simulink model "bench"  (R2025b)
settings: Solver=ode4  StartTime=0.0  StopTime=inf  FixedStep=Ts_gcs  RelTol=1e-3
undefined symbols (not defined in the file): quadcop, Ts_gcs
libraries: instrumentseriallib x2, sldrtlib x1
settings Model: DataDictionary=project.sldd  SimulationMode=accelerator  Creator=Nick  LastModifiedBy=Rakete
settings SolverCC: AutoInsertRateTranBlk=on

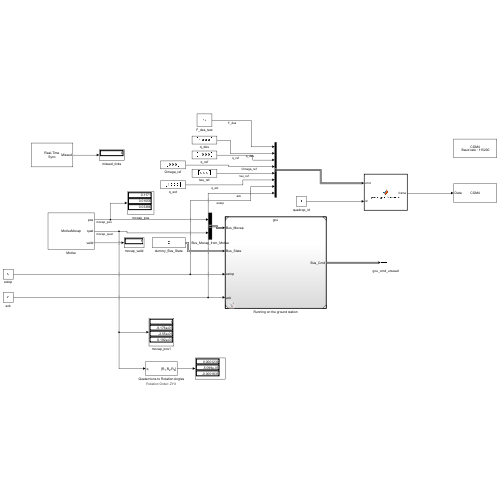
[thumbnail: Simulink's stored preview of the top-level diagram]
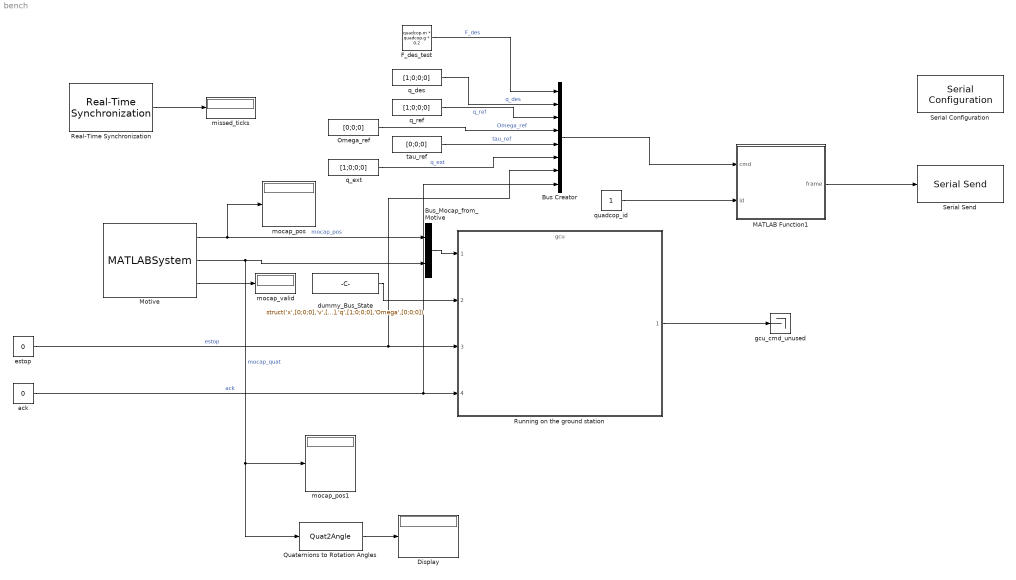
== system bench ==
  Bus Creator : BusCreator  Inputs=8  OutDataTypeStr=Bus: Bus_Cmd
  Bus_Mocap_from_Motive : BusCreator  Inputs=2  OutDataTypeStr=Bus: Bus_Mocap
  Display : Display
  F_des_test : Constant  Value=quadcop.m * quadcop.g * 0.2
  MATLAB Function1 : MATLAB Function  TreatAsAtomicUnit=on
  Motive : MATLABSystem  System=MotiveMocap  HostIP=mocap.host_ip  ClientIP=mocap.client_ip  StreamingID=mocap.streaming_id  SampleTimeSec=Ts_gcs  Verbose=on
      mask Type: MotiveMocap
  Omega_ref : Constant  Value=[0;0;0]
  Quaternions to Rotation Angles : Quat2Angle
      settings: AttributesFormatString=Rotation Order: %<rotationOrder>
  Real-Time Synchronization : sldrtlib/Real-Time Synchronization  SampleTime=Ts_gcs  MaxMissedTicks=inf  ShowMissedTicks=on  YieldWhenWaiting=off
  Running on the ground station : ModelReference  ModelNameDialog=gcu.slx  SimulationMode=Normal  ModelReferenceVersion=1.299
  Serial Configuration : instrumentseriallib/Serial Configuration  Priority=-200000  PortSel=COM4  Port=COM4  ComPort=COM4  BaudRate=115200  DataBits=8  Parity=none  StopBits=1  ByteOrder=little-endian  FlowControl=none  Timeout=10  SimulateUsing=Interpreted execution  BlockInModel=on  aMode=1
      settings: LibrarySourceBlock=c2000lib/Host Communication/Serial Configuration
  Serial Send : instrumentseriallib/Serial Send  Priority=1  PortSel=COM4  Port=COM4  ComPort=COM4  Header=[]  Terminator=<none>  CustomTerminator=[]  EnableBlockingMode=on  SimulateUsing=Interpreted execution  BlockInModel=on  aMode=1
      settings: LibrarySourceBlock=c2000lib/Host Communication/Serial Send
  ack : Constant  Value=0  OutDataTypeStr=boolean
  dummy_Bus_State : Constant  Value=struct('x',[0;0;0],'v',[0;0;0],'q',[1;0;0;0],'Omega',[0;0;0])  OutDataTypeStr=Bus: Bus_State  SampleTime=Ts_gcs
  estop : Constant  Value=0  OutDataTypeStr=uint8
  gcu_cmd_unused : Terminator
  missed_ticks : Display
  mocap_pos : Display
  mocap_pos1 : Display
  mocap_valid : Display
  q_des : Constant  Value=[1;0;0;0]
  q_ext : Constant  Value=[1;0;0;0]
  q_ref : Constant  Value=[1;0;0;0]
  quadcop_id : Constant  OutDataTypeStr=uint8
  tau_ref : Constant  Value=[0;0;0]
  wires:
  Real-Time Synchronization/1 -> missed_ticks/1
  estop/1 -> Bus Creator/7, Running on the ground station/3  "estop"
  ack/1 -> Bus Creator/8, Running on the ground station/4  "ack"
  quadcop_id/1 -> MATLAB Function1/2(id)
  MATLAB Function1/1(frame) -> Serial Send/1
  F_des_test/1 -> Bus Creator/1  "F_des"
  q_des/1 -> Bus Creator/2  "q_des"
  q_ref/1 -> Bus Creator/3  "q_ref"
  Omega_ref/1 -> Bus Creator/4  "Omega_ref"
  tau_ref/1 -> Bus Creator/5  "tau_ref"
  q_ext/1 -> Bus Creator/6  "q_ext"
  Bus Creator/1 -> MATLAB Function1/1(cmd)
  dummy_Bus_State/1 -> Running on the ground station/2
  Running on the ground station/1 -> gcu_cmd_unused/1
  Motive/1 -> mocap_pos/1, Bus_Mocap_from_Motive/1  "mocap_pos"
  Motive/2 -> Quaternions to Rotation Angles/1, mocap_pos1/1, Bus_Mocap_from_Motive/2  "mocap_quat"
  Bus_Mocap_from_Motive/1 -> Running on the ground station/1
  Motive/3 -> mocap_valid/1
  Quaternions to Rotation Angles/1 -> Display/1

== matlab function bench/MATLAB Function1 ==
  data: cmd input Bus: Bus_Cmd; frame output uint8 size=[1 82]; id input uint8 size=[1 1]
function frame = pack_gcs_frame_sl(cmd, id)
%#codegen
% WRAPPER — haelt KEINE Logik. Single Source of Truth ist
% scripts\functions\pack_gcs_frame.m; dieser Block ruft sie nur auf.
% Grund: .slx ist binaer -> Inline-Kopien driften unbemerkt und sind im
% git-Diff unsichtbar (Session 9: 2 von 11 Bloecken waren abgewichen).
% Name MUSS abweichen (_sl), sonst schattet er die externe Funktion.
frame = pack_gcs_frame(cmd, id);
end
